simulink model "model1"  (R2024b)
settings: Solver=VariableStepAuto  StartTime=0.0  StopTime=0.1  MaxStep=1e-3  RelTol=1e-3
undefined symbols (not defined in the file or in its folder): A, Bw, C, Dw, L, Pival, Pival_Dw
settings Model: Creator=Mehmet  LastModifiedBy=Mehmet

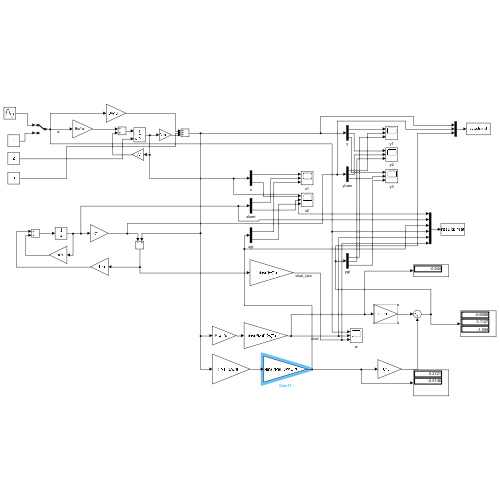
[thumbnail: Simulink's stored preview of the top-level diagram]
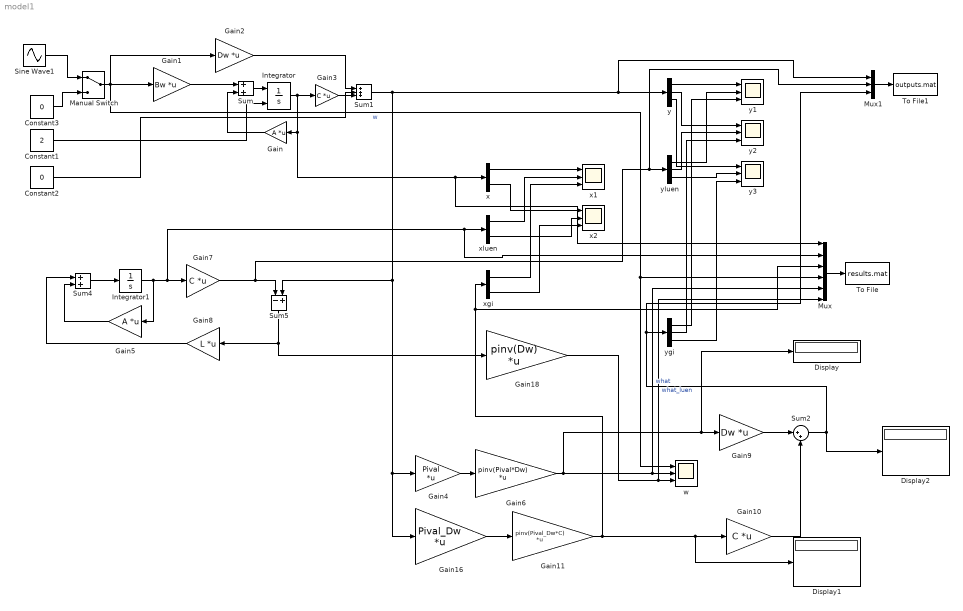
== system model1 ==
  Constant1 : Constant  Value=2
  Constant2 : Constant  Value=0
  Constant3 : Constant  Value=0
  Display : Display
  Display1 : Display
  Display2 : Display
  Gain : Gain  Gain=A  Multiplication=Matrix(K*u)
  Gain1 : Gain  Gain=Bw  Multiplication=Matrix(K*u)
  Gain10 : Gain  Gain=C  Multiplication=Matrix(K*u)
  Gain11 : Gain  Gain=pinv(Pival_Dw*C)  Multiplication=Matrix(K*u)
  Gain16 : Gain  Gain=Pival_Dw  Multiplication=Matrix(K*u)
  Gain18 : Gain  Gain=pinv(Dw)  Multiplication=Matrix(K*u)
  Gain2 : Gain  Gain=Dw  Multiplication=Matrix(K*u)
  Gain3 : Gain  Gain=C  Multiplication=Matrix(K*u)
  Gain4 : Gain  Gain=Pival  Multiplication=Matrix(K*u)
  Gain5 : Gain  Gain=A  Multiplication=Matrix(K*u)
  Gain6 : Gain  Gain=pinv(Pival*Dw)  Multiplication=Matrix(K*u)
  Gain7 : Gain  Gain=C  Multiplication=Matrix(K*u)
  Gain8 : Gain  Gain=L  Multiplication=Matrix(K*u)
  Gain9 : Gain  Gain=Dw  Multiplication=Matrix(K*u)
  Integrator : Integrator  InitialConditionSource=external
  Integrator1 : Integrator
  Manual Switch : ManualSwitch
  Mux : Mux  Inputs=6
  Mux1 : Mux  Inputs=3
  Sine Wave1 : Sin  Frequency=100  SampleTime=0
  Sum : Sum
  Sum1 : Sum  Inputs=+++
  Sum2 : Sum  Inputs=|++
  Sum4 : Sum
  Sum5 : Sum  Inputs=-+
  To File : ToFile  Filename=results.mat  MatrixName=data
  To File1 : ToFile  Filename=outputs.mat  MatrixName=data
  w : Scope  NumInputPorts=3
  x : Demux  Outputs=2
  x1 : Scope  NumInputPorts=3
  x2 : Scope  NumInputPorts=3
  xgi : Demux  Outputs=2
  xluen : Demux  Outputs=2
  y : Demux  Outputs=3
  y1 : Scope  NumInputPorts=3
  y2 : Scope  NumInputPorts=3
  y3 : Scope  NumInputPorts=3
  ygi : Demux  Outputs=3
  yluen : Demux  Outputs=3
  wires:
  Gain/1 -> Sum/2
  Sum/1 -> Integrator/1
  Integrator/1 -> Mux/1, x/1, Gain/1, Gain3/1
  Gain1/1 -> Sum/1
  Gain3/1 -> Sum1/2
  Gain2/1 -> Sum1/1
  Manual Switch/1 -> w/1, Mux/4, Gain2/1, Gain1/1  "w"
  Constant1/1 -> Integrator/2
  Sum4/1 -> Integrator1/1
  Integrator1/1 -> Gain7/1, Mux/2, xluen/1, Gain5/1
  Gain5/1 -> Sum4/2
  Gain7/1 -> Mux1/2, yluen/1, Sum5/1
  Sum5/1 -> Gain18/1, Gain8/1
  Gain8/1 -> Sum4/1
  xluen/1 -> x1/2
  x/2 -> x2/1
  xluen/2 -> x2/2
  Sine Wave1/1 -> Manual Switch/1
  Constant3/1 -> Manual Switch/2
  xgi/1 -> x1/3
  xgi/2 -> x2/3
  Gain6/1 -> Mux/5, w/2, Display/1, Gain9/1  "what"
  y/1 -> y1/1
  yluen/1 -> y1/2
  ygi/1 -> y1/3
  Gain4/1 -> Gain6/1
  y/2 -> y2/1
  yluen/2 -> y2/2
  ygi/2 -> y2/3
  y/3 -> y3/1
  yluen/3 -> y3/2
  ygi/3 -> y3/3
  Gain18/1 -> Mux/6, w/3  "what_luen"
  Constant2/1 -> Sum1/3
  Mux/1 -> To File/1
  Mux1/1 -> To File1/1
  Sum1/1 -> Mux1/1, y/1, Gain16/1, Gain4/1, Sum5/2
  x/1 -> x1/1
  Gain11/1 -> Display1/1, Gain10/1, xgi/1, Mux/3
  Gain9/1 -> Sum2/1
  Gain10/1 -> Sum2/2
  Sum2/1 -> Mux1/3, ygi/1, Display2/1
  Gain16/1 -> Gain11/1
